simulink model "passive_balancing_system"  (R2021b)
settings: Solver=daessc  StartTime=0.0  StopTime=StopTime  MaxStep=0.5  RelTol=1e-3  AbsTol=1e-3
values from neighbouring files (symbols this model uses):
  initial_SOC : value not decoded    [passive_balancing_data.sldd]
  input_current = 0.8    [passive_balancing_data.sldd]
libraries: fl_lib x6, passive_balancing_plant_lib x3, nesl_utility x2
settings Model: DataDictionary=passive_balancing_data.sldd  Creator=tshintai  LastModifiedBy=tshintai
settings SolverCC: AutoScaleAbsTol=off
settings SimscapeCC: SimscapeLogType=all  SimscapeLogToSDI=on  SimscapeLogLimitData=off

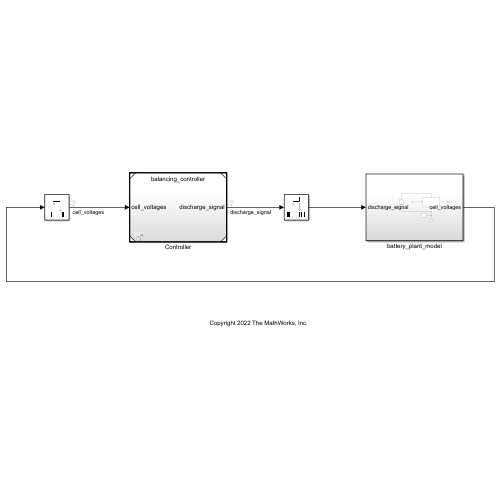
[thumbnail: Simulink's stored preview of the top-level diagram]
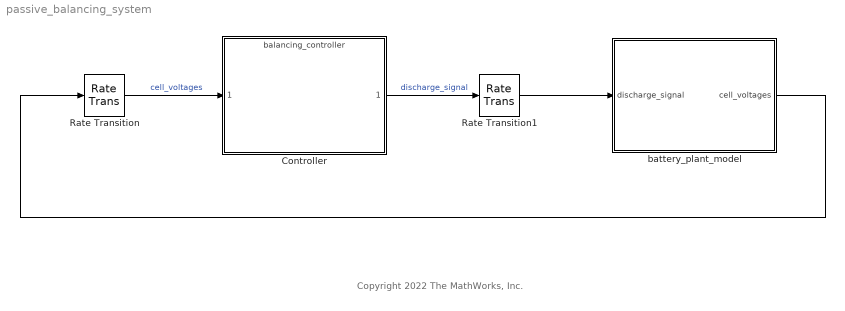
== system passive_balancing_system ==
  note: Copyright 2022 The MathWorks, Inc.
  Controller : ModelReference  ModelNameDialog=balancing_controller  SimulationMode=Normal  ModelReferenceVersion=1.59
  Rate Transition : RateTransition
  Rate Transition1 : RateTransition
  battery_plant_model : Subsystem
  wires:
  battery_plant_model/1(cell_voltages) -> Rate Transition/1
  Controller/1 -> Rate Transition1/1  "discharge_signal"
  Rate Transition/1 -> Controller/1  "cell_voltages"
  Rate Transition1/1 -> battery_plant_model/1(discharge_signal)

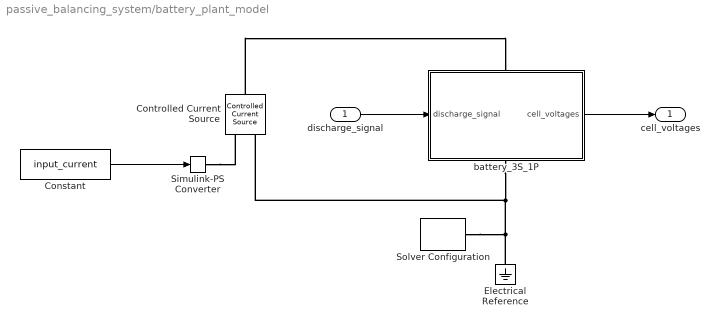
== system passive_balancing_system/battery_plant_model ==
  discharge_signal : Inport
  Constant : Constant  Value=input_current
  Controlled Current Source : fl_lib/Electrical/Electrical Sources/Controlled Current Source
  Electrical Reference : fl_lib/Electrical/Electrical Elements/Electrical Reference
  Simulink-PS Converter : nesl_utility/Simulink-PS Converter  PhysicalDomain=network_engine_domain  SubClassName=ps_input  LeftPortType=input  RightPortType=output  PseudoPeriodic=off  Frequencies=[]  NoiseDistribution=none  NoiseParameters=[]  Unit=1  AffineConversion=off  FilteringAndDerivatives=provide  SimscapeFilterOrder=1  InputFilterTimeConstant=0.001  UdotUserProvided=0
      settings: SourceProductBaseCode=PW,SS
  Solver Configuration : nesl_utility/Solver Configuration  PhysicalDomain=network_engine_domain  SubClassName=solver  LeftPortType=input  RightPortType=generic  Tones=[]  Harmonics=[]  SimulateNoise=off  Profile=off  UseLocalSampling=off  EnableSwitchedLinearOptims=on  FrequencyDomain=off  UseCCode=off  RelTol=0.001  AbsTol=1e-06  MinStep=1e-09  ToWorkspace=off  RevertToSquareIcSolve=off  NumHomotopyIterations=100  PhasorMode=off  PhasorModeNumHarmonics=1  DoDC=off  ResidualTolerance=1e-09  UseLocalSolver=off  LocalSolverChoice=NE_BACKWARD_EULER_ADVANCER  LocalSolverSampleTime=0.001  DoFixedCost=off  MaxNonlinIter=3  MaxModeIter=2  ComputeImpulses=off  ImpulseIterations=2  LinearAlgebra=auto  EquationFormulation=NE_TIME_EF  DelaysMemoryBudget=1024  AutomaticFiltering=on  FilteringTimeConstant=0.001  PartitionStorageMethod=AS_NEEDED  PartitionMemoryBudget=1024  PartitionMethod=ROBUST
      settings: SourceProductBaseCode=PW,SS
  battery_3S_1P : Subsystem
      settings: PortSchema="{\"entries\":[{\"content\":{\"sides\":[{\"content\":{\"connectorIds\":[\"In1\"]},\"type\":\"ConnectorPlacement.EquallySpacedRectSide\",\"uuid\":\"ee17f04a-029d-4e89-9e3a-ff1646692628\"},{\"content\":{\"connectorIds\":[\"Out1\"],\"side\":\"RIGHT\"},\"type\":\"ConnectorPlacement.EquallySpacedRectSide\",\"uuid\":\"2399abcc-b526-417d-8579-01cd22ba38ac\"},{\"content\":{\"connectorIds\":[\"LConn1\"],\"side\":\"TOP\"},\"type\":\"ConnectorPlacement.EquallySpacedRectSide\",\"uuid\":\"d8c78c3d-8a83-4776-bf6f-2f0919d686e9\"},{\"content\":{\"connectorIds\":[\"RConn1\"],\"side\":\"BOTTOM\"},\"type\":\"ConnectorPlacement.EquallySpacedRectSide\",\"uuid\":\"2f75b692-74e5-4d63-8645-63d40a8531e0\"}]},\"type\":\"ConnectorPlacement.EquallySpacedConnector\",\"uuid\":\"f351c746-ad0d-4464-96d4-17f1240d74b6\"}],\"packageUris\":[\"http://schema.mathworks.com/mf0/Connector/R2020b\"],\"version\":\"1.0\"}"
  cell_voltages : Outport
  wires:
  discharge_signal/1 -> battery_3S_1P/1(discharge_signal)
  battery_3S_1P/1(cell_voltages) -> cell_voltages/1
  Constant/1 -> Simulink-PS Converter/1
  connections:
  Simulink-PS Converter/RConn1 -- Controlled Current Source/RConn1
  Solver Configuration/RConn1 -- Electrical Reference/LConn1 -- battery_3S_1P/RConn1 -- Controlled Current Source/RConn2
  Controlled Current Source/LConn1 -- battery_3S_1P/LConn1

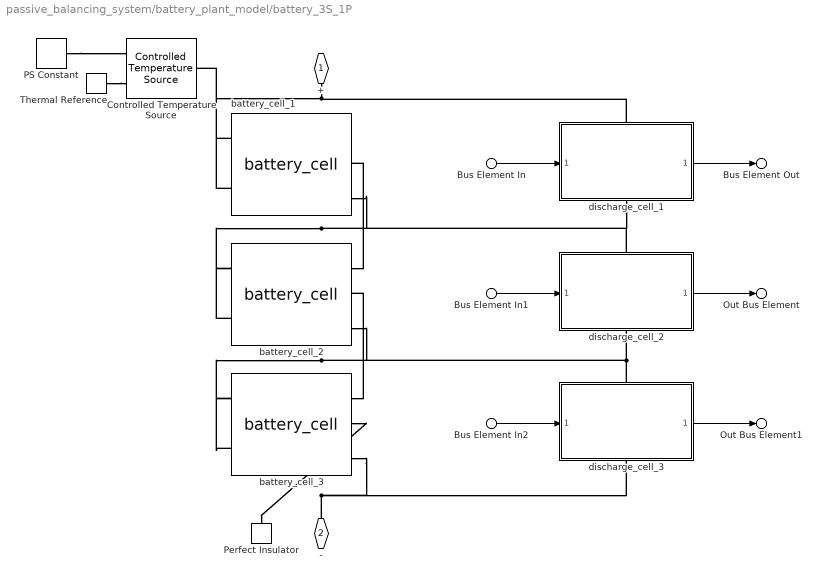
== system passive_balancing_system/battery_plant_model/battery_3S_1P ==
  Bus Element In : Inport  PortName=discharge_signal  Element=s1
  Bus Element In1 : Inport  PortName=discharge_signal  Element=s2
  Bus Element In2 : Inport  PortName=discharge_signal  Element=s3
  Controlled Temperature Source : fl_lib/Thermal/Thermal Sources/Controlled Temperature Source
  PS Constant : fl_lib/Physical Signals/Sources/PS Constant  constant=ambient_temperature
  Perfect Insulator : fl_lib/Thermal/Thermal Elements/Perfect Insulator  T_specify=off  T_priority=None  T=0 K  T_nominal_specify=off  T_nominal_unit=K  T_nominal_value=1
  Thermal Reference : fl_lib/Thermal/Thermal Elements/Thermal Reference
  battery_cell_1 : passive_balancing_plant_lib/battery_cell  SOC_LUT=SOC_LUT  Temperature_LUT=Temperature_LUT  Em_LUT=Em_LUT  R0_LUT=R0_LUT  Capacity_LUT=Capacity_LUT  R1_LUT=R1_LUT  C1_LUT=C1_LUT  cell_mass=cell_mass  cell_Cp_heat=cell_Cp_heat  initial_SOC=initial_SOC(1)  initial_temperature=initial_temperature  cell_area=cell_area  h_conv=h_conv
  battery_cell_2 : passive_balancing_plant_lib/battery_cell  SOC_LUT=SOC_LUT  Temperature_LUT=Temperature_LUT  Em_LUT=Em_LUT  R0_LUT=R0_LUT  Capacity_LUT=Capacity_LUT  R1_LUT=R1_LUT  C1_LUT=C1_LUT  cell_mass=cell_mass  cell_Cp_heat=cell_Cp_heat  initial_SOC=initial_SOC(2)  initial_temperature=initial_temperature  cell_area=cell_area  h_conv=h_conv
  battery_cell_3 : passive_balancing_plant_lib/battery_cell  SOC_LUT=SOC_LUT  Temperature_LUT=Temperature_LUT  Em_LUT=Em_LUT  R0_LUT=R0_LUT  Capacity_LUT=Capacity_LUT  R1_LUT=R1_LUT  C1_LUT=C1_LUT  cell_mass=cell_mass  cell_Cp_heat=cell_Cp_heat  initial_SOC=initial_SOC(3)  initial_temperature=initial_temperature  cell_area=cell_area  h_conv=h_conv
  discharge_cell_1 : Subsystem  ReferencedSubsystem=discharge_cell
      settings: PortSchema="{\"entries\":[{\"content\":{\"sides\":[{\"content\":{\"connectorIds\":[\"In1\"]},\"type\":\"ConnectorPlacement.EquallySpacedRectSide\",\"uuid\":\"27fa656d-5e76-4de7-8620-0e40310d36a8\"},{\"content\":{\"connectorIds\":[\"Out1\"],\"side\":\"RIGHT\"},\"type\":\"ConnectorPlacement.EquallySpacedRectSide\",\"uuid\":\"8322fb78-9706-4b31-a909-8c29c71778d7\"},{\"content\":{\"connectorIds\":[\"LConn1\"],\"side\":\"TOP\"},\"type\":\"ConnectorPlacement.EquallySpacedRectSide\",\"uuid\":\"6f0d5b70-9ba1-4980-9c6d-57ca86e537cf\"},{\"content\":{\"connectorIds\":[\"RConn1\"],\"side\":\"BOTTOM\"},\"type\":\"ConnectorPlacement.EquallySpacedRectSide\",\"uuid\":\"74050354-5197-4766-988c-92549ba1f087\"}]},\"type\":\"ConnectorPlacement.EquallySpacedConnector\",\"uuid\":\"6279a5f0-7db2-4e71-8027-8c4832c7ac7a\"}],\"packageUris\":[\"http://schema.mathworks.com/mf0/Connector/R2020b\"],\"version\":\"1.0\"}"
  discharge_cell_2 : Subsystem  ReferencedSubsystem=discharge_cell
      settings: PortSchema="{\"entries\":[{\"content\":{\"sides\":[{\"content\":{\"connectorIds\":[\"In1\"]},\"type\":\"ConnectorPlacement.EquallySpacedRectSide\",\"uuid\":\"27fa656d-5e76-4de7-8620-0e40310d36a8\"},{\"content\":{\"connectorIds\":[\"Out1\"],\"side\":\"RIGHT\"},\"type\":\"ConnectorPlacement.EquallySpacedRectSide\",\"uuid\":\"8322fb78-9706-4b31-a909-8c29c71778d7\"},{\"content\":{\"connectorIds\":[\"LConn1\"],\"side\":\"TOP\"},\"type\":\"ConnectorPlacement.EquallySpacedRectSide\",\"uuid\":\"6f0d5b70-9ba1-4980-9c6d-57ca86e537cf\"},{\"content\":{\"connectorIds\":[\"RConn1\"],\"side\":\"BOTTOM\"},\"type\":\"ConnectorPlacement.EquallySpacedRectSide\",\"uuid\":\"74050354-5197-4766-988c-92549ba1f087\"}]},\"type\":\"ConnectorPlacement.EquallySpacedConnector\",\"uuid\":\"6279a5f0-7db2-4e71-8027-8c4832c7ac7a\"}],\"packageUris\":[\"http://schema.mathworks.com/mf0/Connector/R2020b\"],\"version\":\"1.0\"}"
  discharge_cell_3 : Subsystem  ReferencedSubsystem=discharge_cell
      settings: PortSchema="{\"entries\":[{\"content\":{\"sides\":[{\"content\":{\"connectorIds\":[\"In1\"]},\"type\":\"ConnectorPlacement.EquallySpacedRectSide\",\"uuid\":\"27fa656d-5e76-4de7-8620-0e40310d36a8\"},{\"content\":{\"connectorIds\":[\"Out1\"],\"side\":\"RIGHT\"},\"type\":\"ConnectorPlacement.EquallySpacedRectSide\",\"uuid\":\"8322fb78-9706-4b31-a909-8c29c71778d7\"},{\"content\":{\"connectorIds\":[\"LConn1\"],\"side\":\"TOP\"},\"type\":\"ConnectorPlacement.EquallySpacedRectSide\",\"uuid\":\"6f0d5b70-9ba1-4980-9c6d-57ca86e537cf\"},{\"content\":{\"connectorIds\":[\"RConn1\"],\"side\":\"BOTTOM\"},\"type\":\"ConnectorPlacement.EquallySpacedRectSide\",\"uuid\":\"74050354-5197-4766-988c-92549ba1f087\"}]},\"type\":\"ConnectorPlacement.EquallySpacedConnector\",\"uuid\":\"6279a5f0-7db2-4e71-8027-8c4832c7ac7a\"}],\"packageUris\":[\"http://schema.mathworks.com/mf0/Connector/R2020b\"],\"version\":\"1.0\"}"
  + : PMIOPort  Side=Left
  - : PMIOPort  Port=2  Side=Right
  Bus Element Out : Outport  PortName=cell_voltages  Element=cell_V_1
  Out Bus Element : Outport  PortName=cell_voltages  Element=cell_V_2
  Out Bus Element1 : Outport  PortName=cell_voltages  Element=cell_V_3
  wires:
  Bus Element In/1 -> discharge_cell_1/1
  Bus Element In1/1 -> discharge_cell_2/1
  Bus Element In2/1 -> discharge_cell_3/1
  discharge_cell_1/1 -> Bus Element Out/1
  discharge_cell_2/1 -> Out Bus Element/1
  discharge_cell_3/1 -> Out Bus Element1/1
  connections:
  battery_cell_1/LConn1 -- Controlled Temperature Source/LConn1
  PS Constant/RConn1 -- Controlled Temperature Source/RConn1
  Thermal Reference/LConn1 -- Controlled Temperature Source/RConn2
  battery_cell_2/LConn1 -- battery_cell_1/RConn2
  discharge_cell_1/RConn1 -- discharge_cell_2/LConn1 -- battery_cell_1/RConn3 -- battery_cell_2/LConn2
  battery_cell_3/LConn1 -- battery_cell_2/RConn2
  discharge_cell_3/LConn1 -- discharge_cell_2/RConn1 -- battery_cell_3/LConn2 -- battery_cell_2/RConn3
  battery_cell_3/RConn2 -- Perfect Insulator/LConn1
  +/RConn1 -- discharge_cell_1/LConn1 -- battery_cell_1/LConn2
  -/RConn1 -- battery_cell_3/RConn3 -- discharge_cell_3/RConn1
